simulink model "PackUDP"  (R2018b)
settings: configuration reference "Active" (kept outside this file)
undefined symbols (not defined in the file): db_ID, P_MLOC_NumberOfNoSendFrames, P_MLOC_NumberOfNoSendFramesCL, P_MLOC_NumberOfNoSendFramesStateEstimate, P_MLOC_NumberOfNoSendFramesTG, P_MLOC_NumberOfNoSendFramesV2X, P_MLOC_NumberOfNoSendFramesVLOC, tS, TUMHealthStatus, TUMVehicleState
libraries: simulink x10, etargetslib x6
settings Model: DataDictionary=PackUDP.sldd  sg_rtwmakecfg_data=_sg_IO821__sglibc_  Creator=lab1  LastModifiedBy=ga25xiw

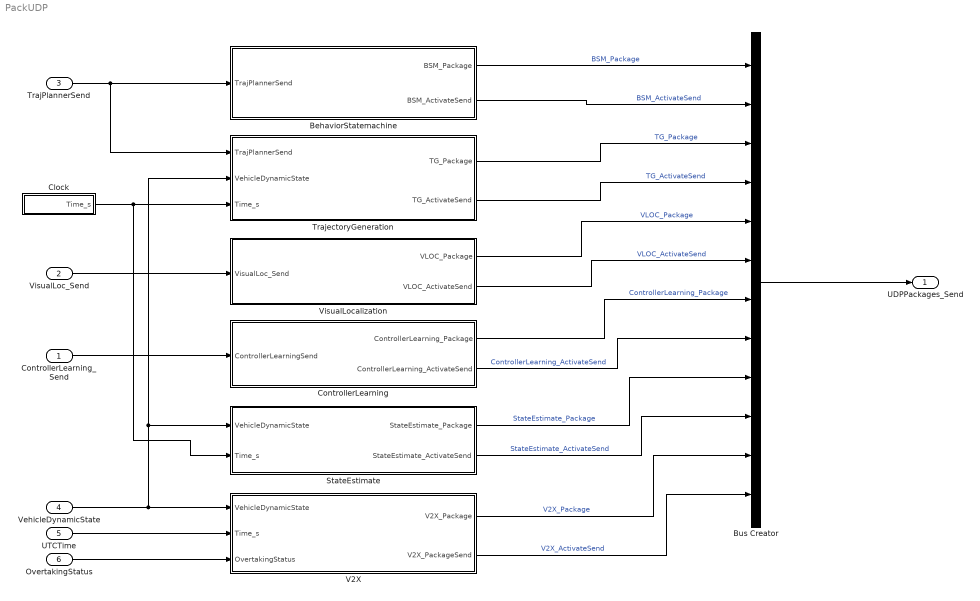
== system PackUDP ==
  ControllerLearning_Send : Inport  OutDataTypeStr=Bus: ControllerLearning_Send  SampleTime=tS  BusOutputAsStruct=on
  VisualLoc_Send : Inport  Port=2  OutDataTypeStr=Bus: VisualLoc_Send  SampleTime=tS  BusOutputAsStruct=on
  TrajPlannerSend : Inport  Port=3  OutDataTypeStr=Bus: TrajPlanner_Send  PortDimensions=1  SampleTime=tS  BusOutputAsStruct=on
  VehicleDynamicState : Inport  Port=4  OutDataTypeStr=Bus: VehicleDynamicState  SampleTime=tS  BusOutputAsStruct=on
  UTCTime : Inport  Port=5  PortDimensions=1
  OvertakingStatus : Inport  Port=6  OutDataTypeStr=uint8  PortDimensions=1
  BehaviorStatemachine : Subsystem
  Bus Creator : BusCreator  Inputs=12
  Clock : Subsystem
  ControllerLearning : Subsystem
  StateEstimate : Subsystem
  TrajectoryGeneration : Subsystem
  V2X : Subsystem
  VisualLocalization : Subsystem
  UDPPackages_Send : Outport  OutDataTypeStr=Bus: UDPPackages_Send
  wires:
  VehicleDynamicState/1 -> TrajectoryGeneration/2(VehicleDynamicState), StateEstimate/1(VehicleDynamicState), V2X/1(VehicleDynamicState)
  TrajPlannerSend/1 -> TrajectoryGeneration/1(TrajPlannerSend), BehaviorStatemachine/1(TrajPlannerSend)
  VisualLoc_Send/1 -> VisualLocalization/1(VisualLoc_Send)
  BehaviorStatemachine/1(BSM_Package) -> Bus Creator/1  "BSM_Package"
  BehaviorStatemachine/2(BSM_ActivateSend) -> Bus Creator/2  "BSM_ActivateSend"
  TrajectoryGeneration/1(TG_Package) -> Bus Creator/3  "TG_Package"
  TrajectoryGeneration/2(TG_ActivateSend) -> Bus Creator/4  "TG_ActivateSend"
  VisualLocalization/1(VLOC_Package) -> Bus Creator/5  "VLOC_Package"
  VisualLocalization/2(VLOC_ActivateSend) -> Bus Creator/6  "VLOC_ActivateSend"
  Bus Creator/1 -> UDPPackages_Send/1
  ControllerLearning_Send/1 -> ControllerLearning/1(ControllerLearningSend)
  ControllerLearning/1(ControllerLearning_Package) -> Bus Creator/7  "ControllerLearning_Package"
  ControllerLearning/2(ControllerLearning_ActivateSend) -> Bus Creator/8  "ControllerLearning_ActivateSend"
  StateEstimate/2(StateEstimate_ActivateSend) -> Bus Creator/10  "StateEstimate_ActivateSend"
  StateEstimate/1(StateEstimate_Package) -> Bus Creator/9  "StateEstimate_Package"
  V2X/2(V2X_PackageSend) -> Bus Creator/12  "V2X_ActivateSend"
  V2X/1(V2X_Package) -> Bus Creator/11  "V2X_Package"
  Clock/1(Time_s) -> StateEstimate/2(Time_s), TrajectoryGeneration/3(Time_s)
  UTCTime/1 -> V2X/2(Time_s)
  OvertakingStatus/1 -> V2X/3(OvertakingStatus)

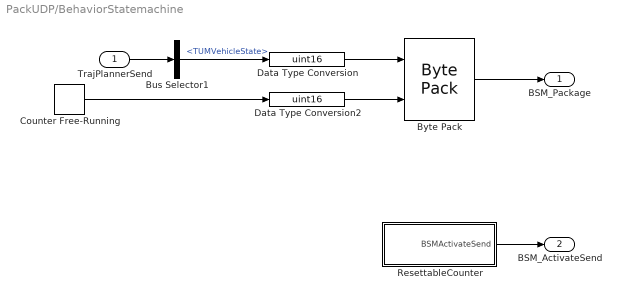
== system PackUDP/BehaviorStatemachine ==
  TrajPlannerSend : Inport
  Bus Selector1 : BusSelector  OutputSignals=TUMVehicleState
  Byte Pack : etargetslib/Byte Pack  datatypes={'uint16', 'uint16'}  byteAlign=1
  Counter Free-Running : simulink/Sources/Counter Free-Running  NumBits=8  tsamp=-1
  Data Type Conversion : DataTypeConversion  OutDataTypeStr=uint16
  Data Type Conversion2 : DataTypeConversion  OutDataTypeStr=uint16
  ResettableCounter : Subsystem
  BSM_Package : Outport
  BSM_ActivateSend : Outport  Port=2
  wires:
  Counter Free-Running/1 -> Data Type Conversion2/1
  Data Type Conversion/1 -> Byte Pack/1
  Data Type Conversion2/1 -> Byte Pack/2
  Byte Pack/1 -> BSM_Package/1
  ResettableCounter/1(BSMActivateSend) -> BSM_ActivateSend/1
  TrajPlannerSend/1 -> Bus Selector1/1
  Bus Selector1/1 -> Data Type Conversion/1  "<TUMVehicleState>"

== system PackUDP/Clock ==
  Counter Free-Running : simulink/Sources/Counter Free-Running  NumBits=32  tsamp=tS
  Data Type Conversion : DataTypeConversion  OutDataTypeStr=double  SaturateOnIntegerOverflow=on
  Gain : Gain  Gain=tS
  Time_s : Outport
  wires:
  Counter Free-Running/1 -> Data Type Conversion/1
  Gain/1 -> Time_s/1
  Data Type Conversion/1 -> Gain/1

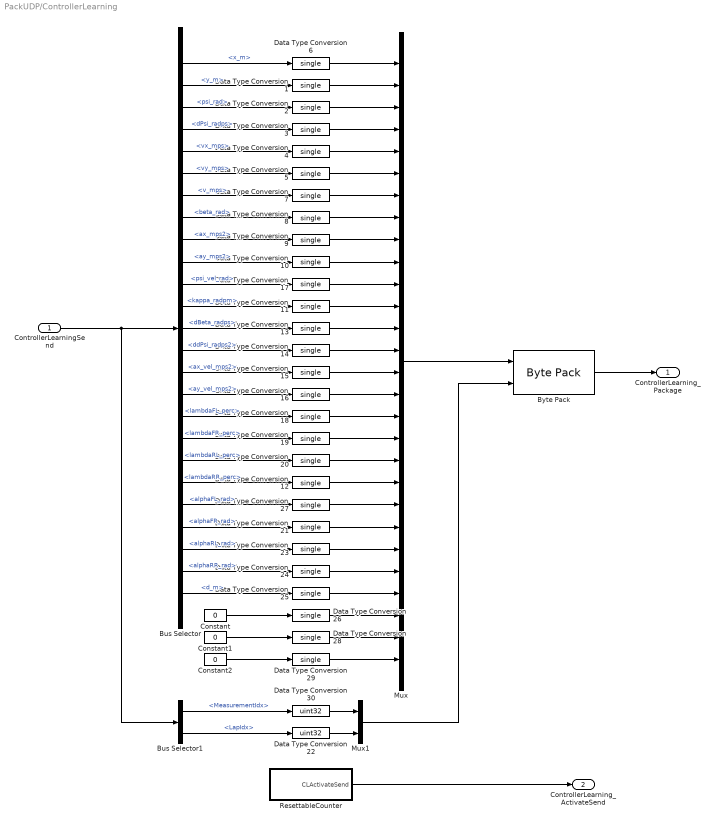
== system PackUDP/ControllerLearning ==
  ControllerLearningSend : Inport
  Bus Selector : BusSelector  OutputSignals=VehicleDynamicState.Pos.x_m,VehicleDynamicState.Pos.y_m,VehicleDynamicState.Pos.psi_rad,VehicleDynamicState.dPsi_radps,VehicleDynamicState.vx_mps,VehicleDynamicState.vy_mps,VehicleDynamicState.v_mps,VehicleDynamicState.beta_rad,VehicleDynamicState.ax_mps2,VehicleDynamicState.ay_mps2,VehicleDynamicState.psi_vel_rad,VehicleDynamicState.kappa_radpm,VehicleDynamicState.dBeta_radps,VehicleDynamicState.ddPsi_radps2,VehicleDynamicState.ax_vel_mps2,VehicleDynamicState.ay_vel_mps2,VehicleDynamicState.lambdaFL_perc,VehicleDynamicState.lambdaFR_perc,VehicleDynamicState.lambdaRL_perc,VehicleDynamicState.lambdaRR_perc,VehicleDynamicState.alphaFL_rad,VehicleDynamicState.alphaFR_rad,VehicleDynamicState.alphaRL_rad,VehicleDynamicState.alphaRR_rad,PathPos.d_m
  Bus Selector1 : BusSelector  OutputSignals=MeasurementIdx,LapIdx
  Byte Pack : etargetslib/Byte Pack  datatypes={'single', 'uint32'}  byteAlign=1
  Constant : Constant  Value=0
  Constant1 : Constant  Value=0
  Constant2 : Constant  Value=0
  Data Type Conversion{1..21,23..29} (28 alike) : DataTypeConversion  OutDataTypeStr=single
  Data Type Conversion22 : DataTypeConversion  OutDataTypeStr=uint32
  Data Type Conversion30 : DataTypeConversion  OutDataTypeStr=uint32
  Mux : Mux  Inputs=28
  Mux1 : Mux  Inputs=2
  ResettableCounter : Subsystem
  ControllerLearning_Package : Outport
  ControllerLearning_ActivateSend : Outport  Port=2
  wires:
  Byte Pack/1 -> ControllerLearning_Package/1
  ResettableCounter/1(CLActivateSend) -> ControllerLearning_ActivateSend/1
  ControllerLearningSend/1 -> Bus Selector1/1, Bus Selector/1
  Bus Selector/1 -> Data Type Conversion6/1  "<x_m>"
  Bus Selector/2 -> Data Type Conversion1/1  "<y_m>"
  Bus Selector/3 -> Data Type Conversion2/1  "<psi_rad>"
  Bus Selector/4 -> Data Type Conversion3/1  "<dPsi_radps>"
  Bus Selector/5 -> Data Type Conversion4/1  "<vx_mps>"
  Bus Selector/6 -> Data Type Conversion5/1  "<vy_mps>"
  Bus Selector/7 -> Data Type Conversion7/1  "<v_mps>"
  Bus Selector/8 -> Data Type Conversion8/1  "<beta_rad>"
  Bus Selector/9 -> Data Type Conversion9/1  "<ax_mps2>"
  Bus Selector/10 -> Data Type Conversion10/1  "<ay_mps2>"
  Bus Selector/11 -> Data Type Conversion17/1  "<psi_vel_rad>"
  Bus Selector/12 -> Data Type Conversion11/1  "<kappa_radpm>"
  Bus Selector/13 -> Data Type Conversion13/1  "<dBeta_radps>"
  Bus Selector/14 -> Data Type Conversion14/1  "<ddPsi_radps2>"
  Bus Selector/15 -> Data Type Conversion15/1  "<ax_vel_mps2>"
  Bus Selector/16 -> Data Type Conversion16/1  "<ay_vel_mps2>"
  Bus Selector/17 -> Data Type Conversion18/1  "<lambdaFL_perc>"
  Bus Selector/18 -> Data Type Conversion19/1  "<lambdaFR_perc>"
  Bus Selector/19 -> Data Type Conversion20/1  "<lambdaRL_perc>"
  Bus Selector/20 -> Data Type Conversion12/1  "<lambdaRR_perc>"
  Bus Selector/21 -> Data Type Conversion27/1  "<alphaFL_rad>"
  Bus Selector/22 -> Data Type Conversion21/1  "<alphaFR_rad>"
  Bus Selector/23 -> Data Type Conversion23/1  "<alphaRL_rad>"
  Bus Selector/24 -> Data Type Conversion24/1  "<alphaRR_rad>"
  Constant/1 -> Data Type Conversion26/1
  Bus Selector1/1 -> Data Type Conversion30/1  "<MeasurementIdx>"
  Data Type Conversion6/1 -> Mux/1
  Data Type Conversion1/1 -> Mux/2
  Data Type Conversion2/1 -> Mux/3
  Data Type Conversion3/1 -> Mux/4
  Data Type Conversion4/1 -> Mux/5
  Data Type Conversion5/1 -> Mux/6
  Data Type Conversion7/1 -> Mux/7
  Data Type Conversion8/1 -> Mux/8
  Data Type Conversion9/1 -> Mux/9
  Data Type Conversion10/1 -> Mux/10
  Data Type Conversion17/1 -> Mux/11
  Data Type Conversion11/1 -> Mux/12
  Data Type Conversion13/1 -> Mux/13
  Data Type Conversion14/1 -> Mux/14
  Data Type Conversion15/1 -> Mux/15
  Data Type Conversion16/1 -> Mux/16
  Data Type Conversion18/1 -> Mux/17
  Data Type Conversion19/1 -> Mux/18
  Data Type Conversion20/1 -> Mux/19
  Data Type Conversion12/1 -> Mux/20
  Data Type Conversion27/1 -> Mux/21
  Data Type Conversion21/1 -> Mux/22
  Data Type Conversion23/1 -> Mux/23
  Data Type Conversion24/1 -> Mux/24
  Data Type Conversion25/1 -> Mux/25
  Data Type Conversion26/1 -> Mux/26
  Data Type Conversion28/1 -> Mux/27
  Data Type Conversion29/1 -> Mux/28
  Mux/1 -> Byte Pack/1
  Bus Selector1/2 -> Data Type Conversion22/1  "<LapIdx>"
  Data Type Conversion30/1 -> Mux1/1
  Data Type Conversion22/1 -> Mux1/2
  Mux1/1 -> Byte Pack/2
  Bus Selector/25 -> Data Type Conversion25/1  "<d_m>"
  Constant1/1 -> Data Type Conversion28/1
  Constant2/1 -> Data Type Conversion29/1

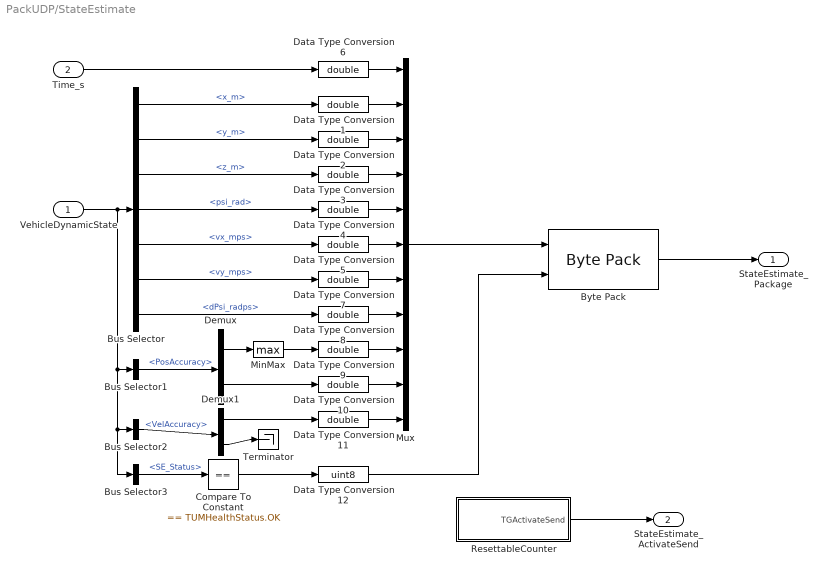
== system PackUDP/StateEstimate ==
  VehicleDynamicState : Inport
  Time_s : Inport  Port=2
  Bus Selector : BusSelector  OutputSignals=Pos.x_m,Pos.y_m,z_m,Pos.psi_rad,vx_mps,vy_mps,dPsi_radps
  Bus Selector1 : BusSelector  OutputSignals=PosAccuracy
  Bus Selector2 : BusSelector  OutputSignals=VelAccuracy
  Bus Selector3 : BusSelector  OutputSignals=SE_Status
  Byte Pack : etargetslib/Byte Pack  datatypes={'double', 'uint8'}  byteAlign=1
  Compare To Constant : simulink/Logic and Bit Operations/Compare To Constant  relop===  const=TUMHealthStatus.OK  OutDataTypeStr=boolean
  Data Type Conversion{1..11} (11 alike) : DataTypeConversion  OutDataTypeStr=double
  Data Type Conversion12 : DataTypeConversion  OutDataTypeStr=uint8
  Demux : Demux  Outputs=[2 1]
  Demux1 : Demux  Outputs=[1 2]
  MinMax : MinMax  Function=max
  Mux : Mux  Inputs=11
  ResettableCounter : Subsystem
  Terminator : Terminator
  StateEstimate_Package : Outport
  StateEstimate_ActivateSend : Outport  Port=2
  wires:
  Data Type Conversion6/1 -> Mux/1
  Data Type Conversion4/1 -> Mux/5
  Data Type Conversion5/1 -> Mux/6
  Data Type Conversion2/1 -> Mux/3
  Data Type Conversion1/1 -> Mux/2
  Data Type Conversion3/1 -> Mux/4
  Time_s/1 -> Data Type Conversion6/1
  VehicleDynamicState/1 -> Bus Selector3/1, Bus Selector2/1, Bus Selector1/1, Bus Selector/1
  Byte Pack/1 -> StateEstimate_Package/1
  Bus Selector/1 -> Data Type Conversion1/1  "<x_m>"
  Bus Selector/2 -> Data Type Conversion2/1  "<y_m>"
  ResettableCounter/1(TGActivateSend) -> StateEstimate_ActivateSend/1
  Data Type Conversion7/1 -> Mux/7
  Data Type Conversion8/1 -> Mux/8
  Data Type Conversion9/1 -> Mux/9
  Data Type Conversion10/1 -> Mux/10
  Data Type Conversion11/1 -> Mux/11
  Bus Selector/3 -> Data Type Conversion3/1  "<z_m>"
  Bus Selector/4 -> Data Type Conversion4/1  "<psi_rad>"
  Bus Selector/5 -> Data Type Conversion5/1  "<vx_mps>"
  Bus Selector/6 -> Data Type Conversion7/1  "<vy_mps>"
  Bus Selector/7 -> Data Type Conversion8/1  "<dPsi_radps>"
  Bus Selector1/1 -> Demux/1  "<PosAccuracy>"
  MinMax/1 -> Data Type Conversion9/1
  Demux/1 -> MinMax/1
  Demux/2 -> Data Type Conversion10/1
  Bus Selector2/1 -> Demux1/1  "<VelAccuracy>"
  Demux1/1 -> Data Type Conversion11/1
  Demux1/2 -> Terminator/1
  Data Type Conversion12/1 -> Byte Pack/2
  Mux/1 -> Byte Pack/1
  Bus Selector3/1 -> Compare To Constant/1  "<SE_Status>"
  Compare To Constant/1 -> Data Type Conversion12/1

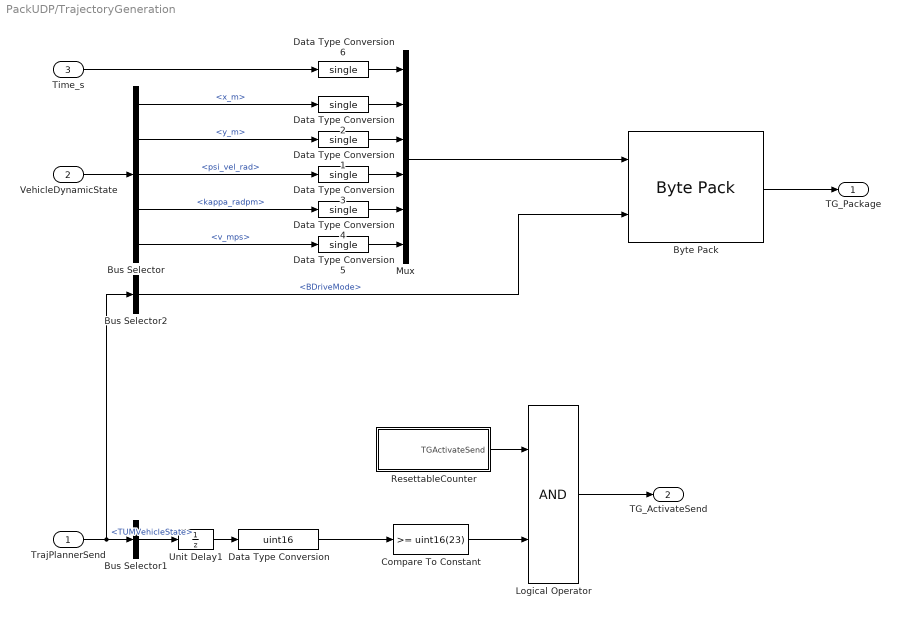
== system PackUDP/TrajectoryGeneration ==
  TrajPlannerSend : Inport
  VehicleDynamicState : Inport  Port=2
  Time_s : Inport  Port=3
  Bus Selector : BusSelector  OutputSignals=Pos.x_m,Pos.y_m,psi_vel_rad,kappa_radpm,v_mps
  Bus Selector1 : BusSelector  OutputSignals=TUMVehicleState
  Bus Selector2 : BusSelector  OutputSignals=BDriveMode
  Byte Pack : etargetslib/Byte Pack  datatypes={'single', 'uint8'}  byteAlign=1
  Compare To Constant : simulink/Logic and Bit Operations/Compare To Constant  relop=>=  const=uint16(23)  OutDataTypeStr=boolean
  Data Type Conversion : DataTypeConversion  OutDataTypeStr=uint16
  Data Type Conversion{1..6} (6 alike) : DataTypeConversion  OutDataTypeStr=single
  Logical Operator : Logic  AllPortsSameDT=off  OutDataTypeStr=boolean
  Mux : Mux  Inputs=6
  ResettableCounter : Subsystem
  Unit Delay1 : UnitDelay  InitialCondition=TUMVehicleState.OFF  SampleTime=tS
  TG_Package : Outport
  TG_ActivateSend : Outport  Port=2
  wires:
  Unit Delay1/1 -> Data Type Conversion/1
  Data Type Conversion/1 -> Compare To Constant/1
  Bus Selector/5 -> Data Type Conversion5/1  "<v_mps>"
  Data Type Conversion6/1 -> Mux/1
  Data Type Conversion4/1 -> Mux/5
  Data Type Conversion5/1 -> Mux/6
  Data Type Conversion1/1 -> Mux/3
  Data Type Conversion2/1 -> Mux/2
  Data Type Conversion3/1 -> Mux/4
  Time_s/1 -> Data Type Conversion6/1
  VehicleDynamicState/1 -> Bus Selector/1
  Mux/1 -> Byte Pack/1
  Bus Selector/4 -> Data Type Conversion4/1  "<kappa_radpm>"
  Byte Pack/1 -> TG_Package/1
  Bus Selector/1 -> Data Type Conversion2/1  "<x_m>"
  Bus Selector/2 -> Data Type Conversion1/1  "<y_m>"
  Bus Selector/3 -> Data Type Conversion3/1  "<psi_vel_rad>"
  Compare To Constant/1 -> Logical Operator/2
  Logical Operator/1 -> TG_ActivateSend/1
  ResettableCounter/1(TGActivateSend) -> Logical Operator/1
  TrajPlannerSend/1 -> Bus Selector2/1, Bus Selector1/1
  Bus Selector1/1 -> Unit Delay1/1  "<TUMVehicleState>"
  Bus Selector2/1 -> Byte Pack/2  "<BDriveMode>"

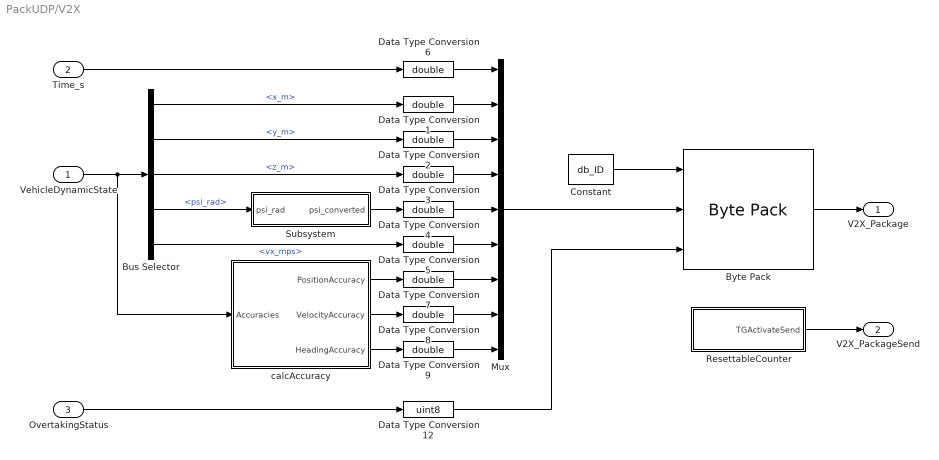
== system PackUDP/V2X ==
  VehicleDynamicState : Inport
  Time_s : Inport  Port=2
  OvertakingStatus : Inport  Port=3
  Bus Selector : BusSelector  OutputSignals=Pos.x_m,Pos.y_m,z_m,Pos.psi_rad,vx_mps
  Byte Pack : etargetslib/Byte Pack  datatypes={'uint16', 'double', 'uint8'}  byteAlign=1
  Constant : Constant  Value=db_ID
  Data Type Conversion{1..9} (9 alike) : DataTypeConversion  OutDataTypeStr=double
  Data Type Conversion12 : DataTypeConversion  OutDataTypeStr=uint8
  Mux : Mux  Inputs=9
  ResettableCounter : Subsystem
  Subsystem : Subsystem
  calcAccuracy : Subsystem
  V2X_Package : Outport
  V2X_PackageSend : Outport  Port=2
  wires:
  Time_s/1 -> Data Type Conversion6/1
  VehicleDynamicState/1 -> calcAccuracy/1(Accuracies), Bus Selector/1
  Byte Pack/1 -> V2X_Package/1
  Bus Selector/1 -> Data Type Conversion1/1  "<x_m>"
  Bus Selector/2 -> Data Type Conversion2/1  "<y_m>"
  ResettableCounter/1(TGActivateSend) -> V2X_PackageSend/1
  Bus Selector/3 -> Data Type Conversion3/1  "<z_m>"
  Bus Selector/5 -> Data Type Conversion5/1  "<vx_mps>"
  Data Type Conversion6/1 -> Mux/1
  Data Type Conversion1/1 -> Mux/2
  Data Type Conversion2/1 -> Mux/3
  Data Type Conversion3/1 -> Mux/4
  Data Type Conversion4/1 -> Mux/5
  Data Type Conversion5/1 -> Mux/6
  Data Type Conversion7/1 -> Mux/7
  Data Type Conversion8/1 -> Mux/8
  Data Type Conversion9/1 -> Mux/9
  Mux/1 -> Byte Pack/2
  Data Type Conversion12/1 -> Byte Pack/3
  Subsystem/1(psi_converted) -> Data Type Conversion4/1
  Bus Selector/4 -> Subsystem/1(psi_rad)  "<psi_rad>"
  calcAccuracy/1(PositionAccuracy) -> Data Type Conversion7/1
  calcAccuracy/2(VelocityAccuracy) -> Data Type Conversion8/1
  calcAccuracy/3(HeadingAccuracy) -> Data Type Conversion9/1
  OvertakingStatus/1 -> Data Type Conversion12/1
  Constant/1 -> Byte Pack/1

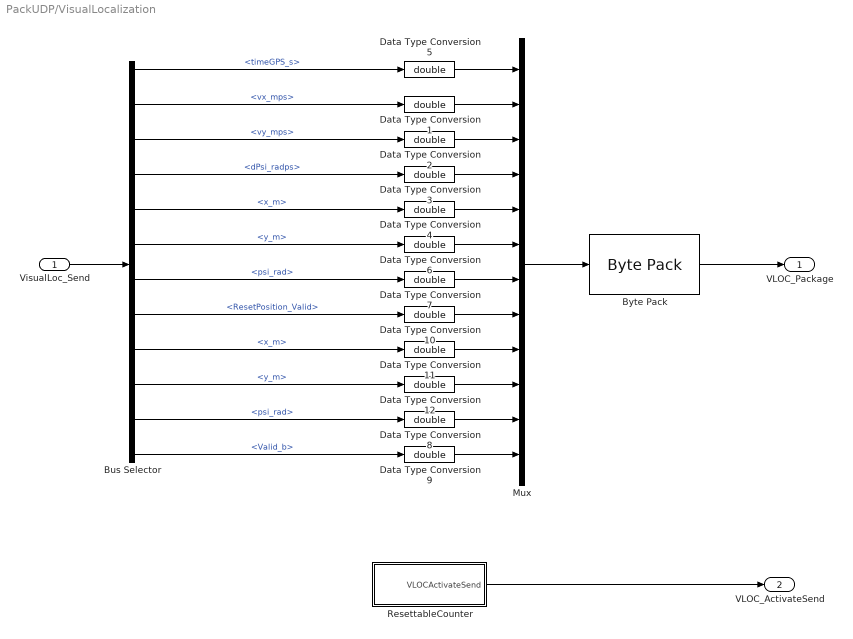
== system PackUDP/VisualLocalization ==
  VisualLoc_Send : Inport
  Bus Selector : BusSelector  OutputSignals=timeGPS_s,vx_mps,vy_mps,dPsi_radps,ResetPosition.x_m,ResetPosition.y_m,ResetPosition.psi_rad,ResetPosition_Valid,Odometry.Position.x_m,Odometry.Position.y_m,Odometry.Position.psi_rad,Odometry.Valid_b
  Byte Pack : etargetslib/Byte Pack  datatypes={'double'}  byteAlign=1
  Data Type Conversion{1..12} (12 alike) : DataTypeConversion  OutDataTypeStr=double
  Mux : Mux  Inputs=12
  ResettableCounter : Subsystem
  VLOC_Package : Outport
  VLOC_ActivateSend : Outport  Port=2
  wires:
  Data Type Conversion5/1 -> Mux/1
  Data Type Conversion4/1 -> Mux/5
  Data Type Conversion6/1 -> Mux/6
  Data Type Conversion2/1 -> Mux/3
  Data Type Conversion1/1 -> Mux/2
  Data Type Conversion3/1 -> Mux/4
  Mux/1 -> Byte Pack/1
  Data Type Conversion7/1 -> Mux/7
  Data Type Conversion8/1 -> Mux/11
  Data Type Conversion10/1 -> Mux/8
  Data Type Conversion11/1 -> Mux/9
  Data Type Conversion12/1 -> Mux/10
  Byte Pack/1 -> VLOC_Package/1
  VisualLoc_Send/1 -> Bus Selector/1
  Bus Selector/3 -> Data Type Conversion2/1  "<vy_mps>"
  Bus Selector/5 -> Data Type Conversion4/1  "<x_m>"
  Bus Selector/6 -> Data Type Conversion6/1  "<y_m>"
  Bus Selector/7 -> Data Type Conversion7/1  "<psi_rad>"
  Bus Selector/9 -> Data Type Conversion11/1  "<x_m>"
  Bus Selector/10 -> Data Type Conversion12/1  "<y_m>"
  Bus Selector/11 -> Data Type Conversion8/1  "<psi_rad>"
  Bus Selector/4 -> Data Type Conversion3/1  "<dPsi_radps>"
  Bus Selector/2 -> Data Type Conversion1/1  "<vx_mps>"
  Bus Selector/1 -> Data Type Conversion5/1  "<timeGPS_s>"
  Bus Selector/8 -> Data Type Conversion10/1  "<ResetPosition_Valid>"
  Data Type Conversion9/1 -> Mux/12
  Bus Selector/12 -> Data Type Conversion9/1  "<Valid_b>"
  ResettableCounter/1(VLOCActivateSend) -> VLOC_ActivateSend/1

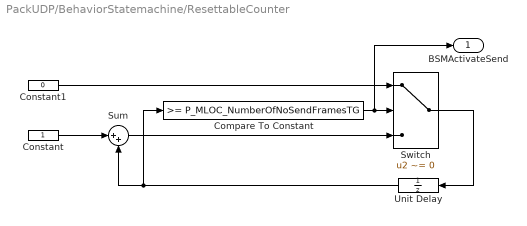
== system PackUDP/BehaviorStatemachine/ResettableCounter ==
  Compare To Constant : simulink/Logic and Bit Operations/Compare To Constant  relop=>=  const=P_MLOC_NumberOfNoSendFramesTG  OutDataTypeStr=boolean
  Constant : Constant
  Constant1 : Constant  Value=0
  Sum : Sum  Inputs=|++
  Switch : Switch  Criteria=u2 ~= 0  Threshold=P_MLOC_NumberOfNoSendFrames
  Unit Delay : UnitDelay  SampleTime=-1
  BSMActivateSend : Outport
  wires:
  Unit Delay/1 -> Compare To Constant/1, Sum/2
  Compare To Constant/1 -> BSMActivateSend/1, Switch/2
  Switch/1 -> Unit Delay/1
  Constant/1 -> Sum/1
  Constant1/1 -> Switch/1
  Sum/1 -> Switch/3

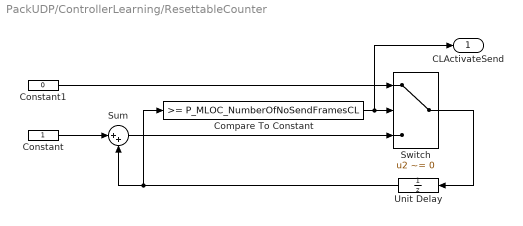
== system PackUDP/ControllerLearning/ResettableCounter ==
  Compare To Constant : simulink/Logic and Bit Operations/Compare To Constant  relop=>=  const=P_MLOC_NumberOfNoSendFramesCL  OutDataTypeStr=boolean
  Constant : Constant
  Constant1 : Constant  Value=0
  Sum : Sum  Inputs=|++
  Switch : Switch  Criteria=u2 ~= 0  Threshold=P_MLOC_NumberOfNoSendFrames
  Unit Delay : UnitDelay  SampleTime=-1
  CLActivateSend : Outport
  wires:
  Unit Delay/1 -> Compare To Constant/1, Sum/2
  Compare To Constant/1 -> CLActivateSend/1, Switch/2
  Switch/1 -> Unit Delay/1
  Constant/1 -> Sum/1
  Constant1/1 -> Switch/1
  Sum/1 -> Switch/3

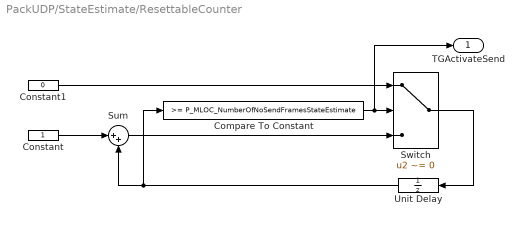
== system PackUDP/StateEstimate/ResettableCounter ==
  Compare To Constant : simulink/Logic and Bit Operations/Compare To Constant  relop=>=  const=P_MLOC_NumberOfNoSendFramesStateEstimate  OutDataTypeStr=boolean
  Constant : Constant
  Constant1 : Constant  Value=0
  Sum : Sum  Inputs=|++
  Switch : Switch  Criteria=u2 ~= 0  Threshold=P_MLOC_NumberOfNoSendFrames
  Unit Delay : UnitDelay  SampleTime=-1
  TGActivateSend : Outport
  wires:
  Unit Delay/1 -> Compare To Constant/1, Sum/2
  Compare To Constant/1 -> TGActivateSend/1, Switch/2
  Switch/1 -> Unit Delay/1
  Constant/1 -> Sum/1
  Constant1/1 -> Switch/1
  Sum/1 -> Switch/3

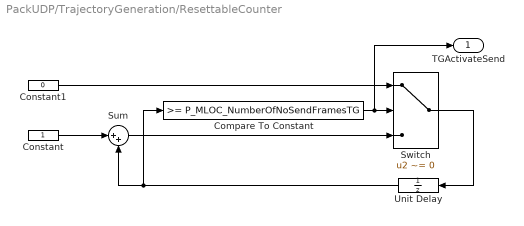
== system PackUDP/TrajectoryGeneration/ResettableCounter ==
  Compare To Constant : simulink/Logic and Bit Operations/Compare To Constant  relop=>=  const=P_MLOC_NumberOfNoSendFramesTG  OutDataTypeStr=boolean
  Constant : Constant
  Constant1 : Constant  Value=0
  Sum : Sum  Inputs=|++
  Switch : Switch  Criteria=u2 ~= 0  Threshold=P_MLOC_NumberOfNoSendFrames
  Unit Delay : UnitDelay  SampleTime=-1
  TGActivateSend : Outport
  wires:
  Unit Delay/1 -> Compare To Constant/1, Sum/2
  Compare To Constant/1 -> TGActivateSend/1, Switch/2
  Switch/1 -> Unit Delay/1
  Constant/1 -> Sum/1
  Constant1/1 -> Switch/1
  Sum/1 -> Switch/3

== system PackUDP/V2X/ResettableCounter ==
  Compare To Constant : simulink/Logic and Bit Operations/Compare To Constant  relop=>=  const=P_MLOC_NumberOfNoSendFramesV2X  OutDataTypeStr=boolean
  Constant : Constant
  Constant1 : Constant  Value=0
  Sum : Sum  Inputs=|++
  Switch : Switch  Criteria=u2 ~= 0  Threshold=P_MLOC_NumberOfNoSendFrames
  Unit Delay : UnitDelay  SampleTime=-1
  TGActivateSend : Outport
  wires:
  Unit Delay/1 -> Compare To Constant/1, Sum/2
  Compare To Constant/1 -> TGActivateSend/1, Switch/2
  Switch/1 -> Unit Delay/1
  Constant/1 -> Sum/1
  Constant1/1 -> Switch/1
  Sum/1 -> Switch/3

== system PackUDP/V2X/Subsystem ==
  psi_rad : Inport
  Constant3 : Constant  Value=2*pi
  Sum : Sum  Inputs=|++
  Switch : Switch  Criteria=u2 > Threshold
  psi_converted : Outport
  wires:
  Sum/1 -> Switch/3
  psi_rad/1 -> Sum/1, Switch/1, Switch/2
  Switch/1 -> psi_converted/1
  Constant3/1 -> Sum/2

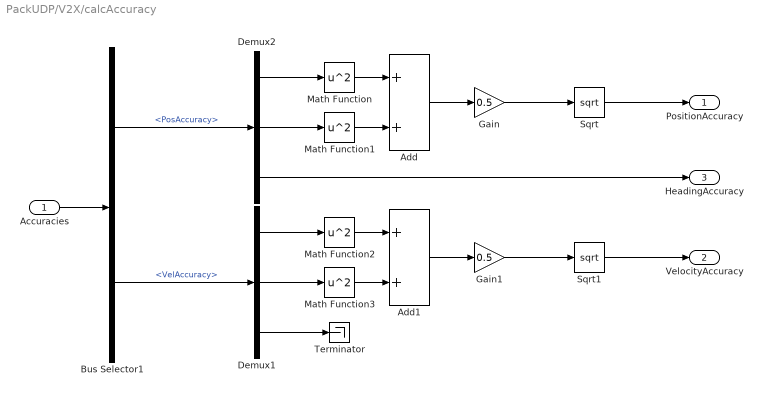
== system PackUDP/V2X/calcAccuracy ==
  Accuracies : Inport
  Add : Sum
  Add1 : Sum
  Bus Selector1 : BusSelector  OutputSignals=PosAccuracy,VelAccuracy
  Demux1 : Demux  Outputs=[1 1 1]
  Demux2 : Demux  Outputs=[1 1 1]
  Gain : Gain  Gain=0.5
  Gain1 : Gain  Gain=0.5
  Math Function{,1..3} (4 alike) : Math  Operator=square  SaturateOnIntegerOverflow=on
  Sqrt : Sqrt  SaturateOnIntegerOverflow=on
  Sqrt1 : Sqrt  SaturateOnIntegerOverflow=on
  Terminator : Terminator
  PositionAccuracy : Outport
  VelocityAccuracy : Outport  Port=2
  HeadingAccuracy : Outport  Port=3
  wires:
  Bus Selector1/1 -> Demux2/1  "<PosAccuracy>"
  Accuracies/1 -> Bus Selector1/1
  Demux2/3 -> HeadingAccuracy/1
  Demux2/2 -> Math Function1/1
  Demux2/1 -> Math Function/1
  Math Function1/1 -> Add/2
  Math Function/1 -> Add/1
  Add/1 -> Gain/1
  Add1/1 -> Gain1/1
  Math Function3/1 -> Add1/2
  Demux1/1 -> Math Function2/1
  Demux1/2 -> Math Function3/1
  Math Function2/1 -> Add1/1
  Bus Selector1/2 -> Demux1/1  "<VelAccuracy>"
  Demux1/3 -> Terminator/1
  Gain/1 -> Sqrt/1
  Sqrt/1 -> PositionAccuracy/1
  Gain1/1 -> Sqrt1/1
  Sqrt1/1 -> VelocityAccuracy/1

== system PackUDP/VisualLocalization/ResettableCounter ==
  Compare To Constant : simulink/Logic and Bit Operations/Compare To Constant  relop=>=  const=P_MLOC_NumberOfNoSendFramesVLOC  OutDataTypeStr=boolean
  Constant : Constant
  Constant1 : Constant  Value=0
  Sum : Sum  Inputs=|++
  Switch : Switch  Criteria=u2 ~= 0  Threshold=P_MLOC_NumberOfNoSendFrames
  Unit Delay : UnitDelay  SampleTime=-1
  VLOCActivateSend : Outport
  wires:
  Unit Delay/1 -> Compare To Constant/1, Sum/2
  Compare To Constant/1 -> VLOCActivateSend/1, Switch/2
  Switch/1 -> Unit Delay/1
  Constant/1 -> Sum/1
  Constant1/1 -> Switch/1
  Sum/1 -> Switch/3
